simulink model "LQG_test"  (R2015a)
settings: Solver=ode5  StartTime=0.0  StopTime=14  FixedStep=1e-4  RelTol=1e-3
values from neighbouring files (symbols this model uses):
  Ak = [-686.540167589 -2525.24249406 3003.88260074 -3376.17154505 -919.51585859 -329.995557257 0.554863416066 -1.08710235968 -676.651099981 -520.714667022 1.21590501094 -2.53862308337 ... (256 elements, 16x16)]    [controller.mat]    (also in main_matlab_step1.m = rlqg.A)
  Ap = Ap(nn-nnn+1:nn,nn-nnn+1:nn)    [main_matlab_step1.m]    (also in plant.mat = [-21.9168905393 -6329.30033318 0 0 0 0 0 0 0 0 0 0 ... (256 )
  Bk = [1.97719987834 -11.3684759745 -9.05802419262 10.0670713674 2.75617939968 0.986945919802 0.000704388812111 0.000546312859848 1.994467134 1.56925194637 -0.000623043221846 -0.000401188810085 ... (16 elements, 16x1)]    [controller.mat]    (also in main_matlab_step1.m = rlqg.B)
  Bpu = Bp(nn-nnn+1:nn,:)    [main_matlab_step1.m]
  Bpw = Hp(nn-nnn+1:nn,:)    [main_matlab_step1.m]
  Ck = [222.229329693 -243.535885757 -178.555900893 231.804330898 -0.516735556885 1.68229660692 1.7803425243 2.91724348036 -1828.17787203 679.97679107 -124.670473614 -98.6387833172 ... (32 elements, 2x16)]    [controller.mat]    (also in main_matlab_step1.m = rlqg.C)
  Cpy = Cp(:,nn-nnn+1:nn)    [main_matlab_step1.m]
  Dk = [0 0]    [controller.mat]    (also in main_matlab_step1.m = rlqg.D)
libraries: simulink x1
settings Model: Creator=p4wp4w  LastModifiedBy=p4wp4w

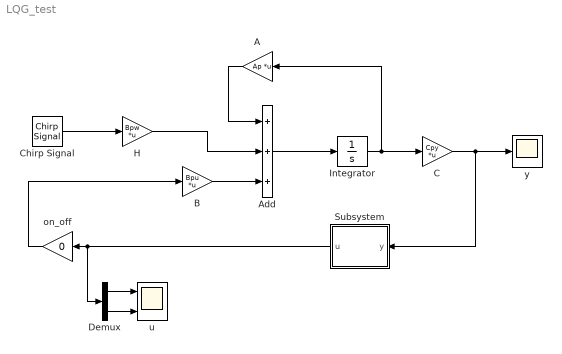
== system LQG_test ==
  A : Gain  Gain=Ap  Multiplication=Matrix(K*u)
  Add : Sum  Inputs=+++
  B : Gain  Gain=Bpu  Multiplication=Matrix(K*u)
  C : Gain  Gain=Cpy  Multiplication=Matrix(K*u)
  Chirp Signal : simulink/Sources/Chirp Signal  f1=0.1  T=14  f2=140
  Demux : Demux  Outputs=2
  H : Gain  Gain=Bpw  Multiplication=Matrix(K*u)
  Integrator : Integrator
  Subsystem : Subsystem
  on_off : Gain  Gain=0
  u : Scope  NumInputPorts=2
      settings: YMin=-5~-5  YMax=5~5
  y : Scope
      settings: YMin=-0.03  YMax=0.03
  wires:
  Add/1 -> Integrator/1
  A/1 -> Add/1
  B/1 -> Add/3
  Integrator/1 -> C/1, A/1
  H/1 -> Add/2
  Chirp Signal/1 -> H/1
  on_off/1 -> B/1
  Demux/1 -> u/1
  Demux/2 -> u/2
  Subsystem/1("u ") -> Demux/1, on_off/1
  C/1 -> Subsystem/1(y), y/1

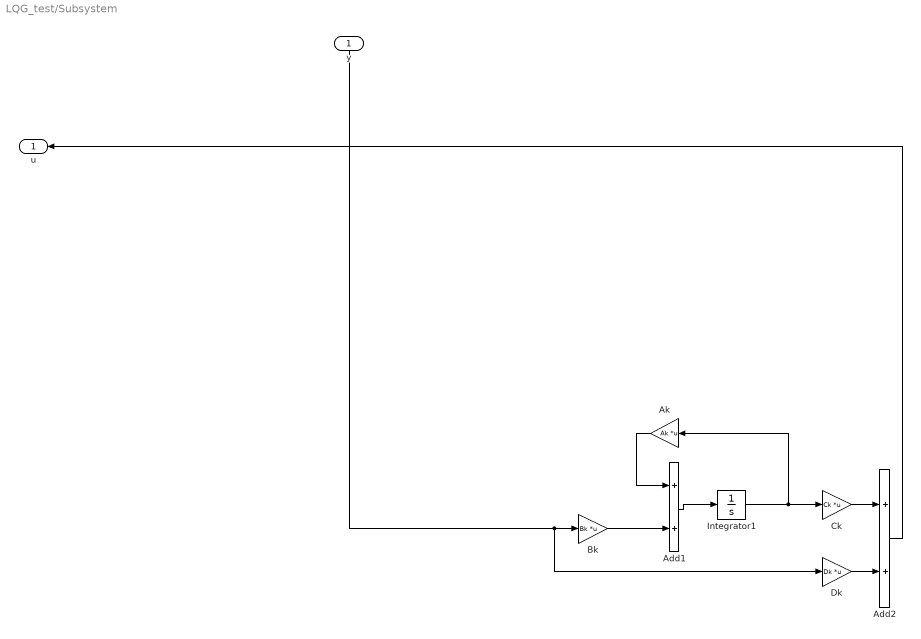
== system LQG_test/Subsystem ==
  y : Inport
  Add1 : Sum
  Add2 : Sum
  Ak : Gain  Gain=Ak  Multiplication=Matrix(K*u)
  Bk : Gain  Gain=Bk  Multiplication=Matrix(K*u)
  Ck : Gain  Gain=Ck  Multiplication=Matrix(K*u)
  Dk : Gain  Gain=Dk  Multiplication=Matrix(K*u)
  Integrator1 : Integrator
  "u " : Outport
  wires:
  y/1 -> Bk/1, Dk/1
  Add2/1 -> "u "/1
  Bk/1 -> Add1/2
  Ak/1 -> Add1/1
  Add1/1 -> Integrator1/1
  Dk/1 -> Add2/2
  Integrator1/1 -> Ck/1, Ak/1
  Ck/1 -> Add2/1
